simulink model "traffic_lights"  (R2021a)
settings: Solver=VariableStepAuto  StartTime=0.0  StopTime=inf  RelTol=1e-3
libraries: vrlib x1
settings Model: Creator=kbhar  LastModifiedBy=kbhar

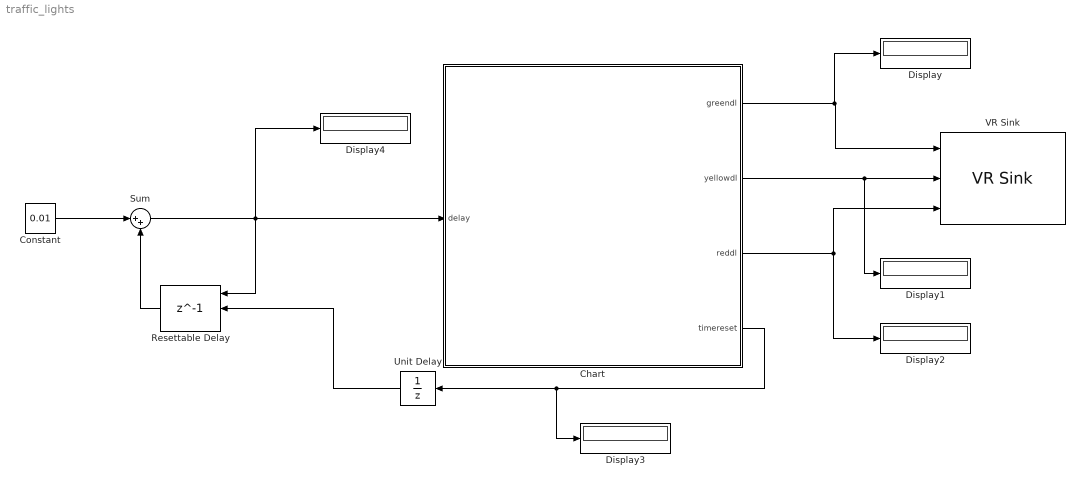
== system traffic_lights ==
  Chart : Stateflow chart  TreatAsAtomicUnit=on
      settings: PortSchema="{\"entries\":[{\"content\":{\"sides\":[{\"content\":{\"connectorIds\":[\"In1\"]},\"type\":\"ConnectorPlacement.EquallySpacedRectSide\",\"uuid\":\"413bb506-1518-4eb7-90cb-7fd0c8a7acea\"},{\"content\":{\"connectorIds\":[\"Out3\",\"Out2\",\"Out1\",\"Out4\"],\"side\":\"RIGHT\"},\"type\":\"ConnectorPlacement.EquallySpacedRectSide\",\"uuid\":\"8cf71874-3035-44ee-8d65-7af52a553ef5\"},{\"content\":{\"connectorIds\":[],\"side\":\"TOP\"},\"type\":\"ConnectorPlacement.EquallySpacedRectSide\",\"uuid\":\"b5cb11e2-d3b0-4c51-9254-bc2ab012951d\"}]},\"type\":\"ConnectorPlacement.EquallySpacedConnector\",\"uuid\":\"4e7be213-afd6-42e5-92c2-a0a83621d821\"}],\"packageUris\":[\"http://schema.mathworks.com/mf0/Connector/R2020b\"],\"version\":\"1.0\"}"
  Constant : Constant  Value=0.01
  Display{,1..4} (5 alike) : Display
  Resettable Delay : Delay  DelayLength=1  InitialConditionSource=Input port  ExternalReset=Rising
      settings: InputPortMap=u0,r5,p4
  Sum : Sum  Inputs=|++
  Unit Delay : UnitDelay  SampleTime=-1  HasFrameUpgradeWarning=on
  VR Sink : vrlib/VR Sink  InstantiateOnLoad=on  SampleTime=0.1  ViewEnable=on  RemoteChange=off  RemoteView=off  FieldsWritten=greendl.on.1.1.1.logical#yellowdl.on.1.1.1.logical#reddl.on.1.1.1.logical  WorldFileName=C:\Bharat\College\Projects\Arm Control\Files\traffic_lights.wrl  AutoView=off  VideoDimensions=[]  AllowVariableSize=off
  wires:
  Chart/1(reddl) -> Display2/1, VR Sink/3
  Chart/2(yellowdl) -> Display1/1, VR Sink/2
  Chart/3(greendl) -> Display/1, VR Sink/1
  Constant/1 -> Sum/1
  Resettable Delay/1 -> Sum/2
  Sum/1 -> Resettable Delay/1, Display4/1, Chart/1(delay)
  Chart/4(timereset) -> Display3/1, Unit Delay/1
  Unit Delay/1 -> Resettable Delay/2

== stateflow chart traffic_lights/Chart ==
  state startstate
    reddl = 0; yellowdl = 0; greendl =0;
    timereset = 0;
  state stopstate
    reddl = 1; yellowdl = 0; greendl =0;
    timereset = 1;
  state waitonestate
    reddl = 0; yellowdl = 1; greendl =0;
    timereset = 0;
  state waittwostate
    reddl = 0; yellowdl = 1; greendl =0;
  state gostate
    reddl = 0; yellowdl = 0; greendl =1;
  (default) -> startstate
  startstate -> stopstate
  waittwostate -> stopstate : [delay > 30]
  stopstate -> waitonestate : [delay > 10]
  waitonestate -> gostate : [delay > 15]
  gostate -> waittwostate : [delay > 25]
  data: delay input; reddl output; yellowdl output; greendl output; timereset output
